simulink model "OLD_slave"  (R2023b)
settings: Solver=VariableStepAuto  StartTime=0.0  StopTime=inf  RelTol=1e-3
settings Model: Creator=sabat  LastModifiedBy=sabat
settings SolverCC: AlgebraicLoopSolver=TrustRegion
settings OptimizationCC: DefaultParameterBehavior=Inlined  EnhancedBackFolding=on  PassReuseOutputArgsAs=Individual arguments  ZeroExternalMemoryAtStartup=off  ZeroInternalMemoryAtStartup=off  OptimizeBlockOrder=speed  DifferentSizesBufferReuse=on  OptimizationCustomize=off  EfficientTunableParamExpr=on
settings DebuggingCC: ParameterTunabilityLossMsg=error
settings SFSimCC: MATLABDynamicMemAlloc=off
settings RTWCC: Description=Embedded Coder  SystemTargetFile=ert.tlc  TemplateMakefile=ert_default_tmf
settings CodeAppCC: ForceParamTrailComments=on  IgnoreCustomStorageClasses=off  OperatorAnnotations=on  SimulinkDataObjDesc=on  SFDataObjDesc=on  InsertBlockDesc=on
settings ERTTargetCC: TargetLangStandard=C99 (ISO)  GenerateSampleERTMain=on  InlinedParameterPlacement=NonHierarchical  ERTCustomFileTemplate=example_file_process.tlc

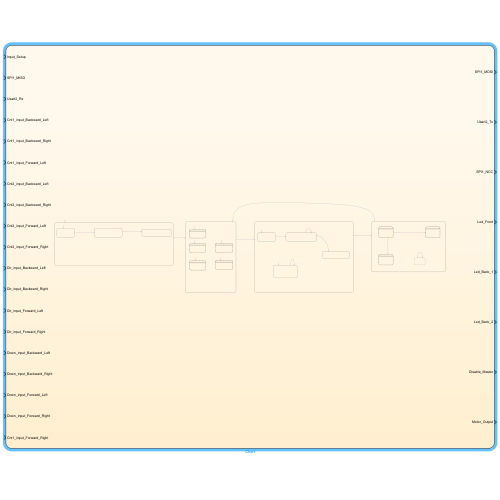
[thumbnail: Simulink's stored preview of the top-level diagram]
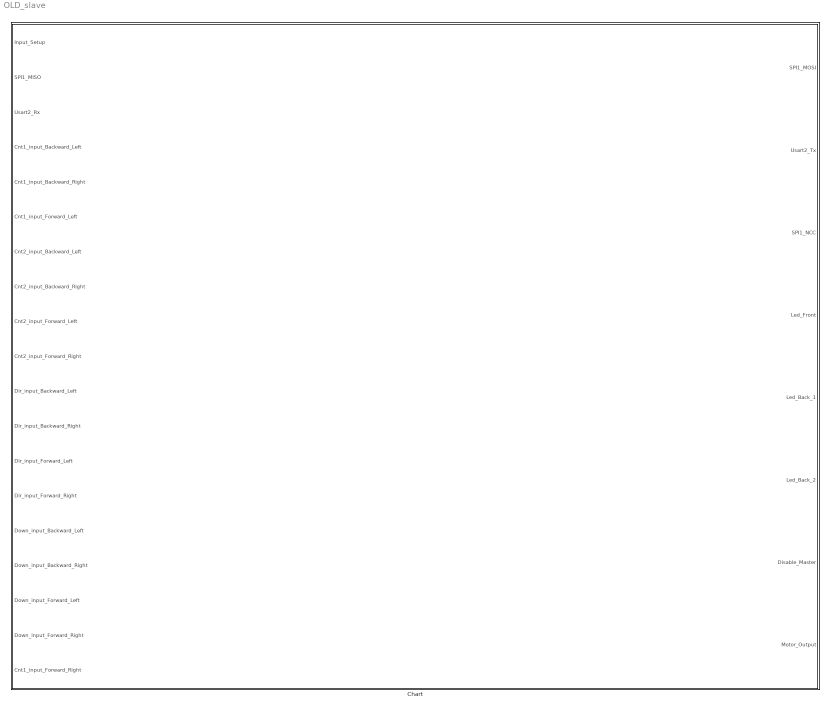
== system OLD_slave ==
  Chart : Stateflow chart  TreatAsAtomicUnit=on

== stateflow chart OLD_slave/Chart ==
  state Read_Inputs_State
    state Logic [parallel]
      settings: executionOrder=1
      state Sensor_Not_Read
      state Sensor_Read
      (default) -> Sensor_Not_Read
      Sensor_Not_Read -> Sensor_Read : [ after(1,Encoder_Backward_Left)   && after(1,Encoder_Backward_Right)  && after(1,Encoder_Forward_Right)  && after(1,Encoder_Forward_Left)  && after(Read_Deadline, msec)]{send(Processing,Read_Inputs_State)}
    state Encoder_Forward_Left [parallel]
      settings: executionOrder=2
      state Read
        cnt2_Forward_Left = Cnt2_input_Forward_Left;
        Dir_Forward_Left = Dir_input_Forward_Left;
        Down_Forward_Left =Down_input_Forward_Left;
        if  Down_Forward_Left
        if (cnt2_Forward_Left < cnt1_Forward_Left)
        diff_Forward_Left = cnt1_Forward_Left - cnt2_Forward_Left;
        else
        diff_Forward_Left = (65535 - cnt2_Forward_Left) + cnt1_Forward_Left;
        end
        else
        if (cnt2_Forward_Left > cnt1_Forward_Left)
        diff _Forward_Left= cnt2_Forward_Left - cnt1_Forward_Left;
        else
        diff _Forward_Left= (65535 - cnt1_Forward_Left) + cnt2_Forward_Left;
        end
        end
        Speed_Forward_Left= diff_Forward_Left / PPR / 60;
      state Start
        cnt1_Forward_Left = Cnt1_input_Forward_Left
      state End
      (default) -> Read_Inputs_State.Encoder_Forward_Left.Start
      Read_Inputs_State.Encoder_Forward_Left.Start -> Read_Inputs_State.Encoder_Forward_Left.Read : [after(300, msec)]
      Read_Inputs_State.Encoder_Forward_Left.Read -> Read_Inputs_State.Encoder_Forward_Left.End : {send(Encoder_Forward_Left,Read_Inputs_State.Logic)}
    state Encoder_Forward_Right [parallel]
      settings: executionOrder=5
      state Read
        cnt2_Forward_Right = Cnt2_input_Forward_Right;
        Dir_Forward_Right = Dir_input_Forward_Right;
        Down_Forward_Right =Down_input_Forward_Right;
        if  Down_Forward_Right
        if (cnt2_Forward_Right < cnt1_Forward_Right)
        diff_Forward_Right = cnt1_Forward_Right - cnt2_Forward_Right;
        else
        diff_Forward_Right = (65535 - cnt2_Forward_Right) + cnt1_Forward_Right;
        end
        else
        if (cnt2_Forward_Right > cnt1_Forward_Right)
        diff _Forward_Right= cnt2_Forward_Right - cnt1_Forward_Right;
        else
        diff _Forward_Right= (65535 - cnt1_Forward_Right) + cnt2_Forward_Right;
        end
        end
        Speed_Forward_Right= diff_Forward_Right / PPR / 60
      state Start
        cnt1_Forward_Right= Cnt1_input_Forward_Right
      state End
      (default) -> Read_Inputs_State.Encoder_Forward_Right.Start
      Read_Inputs_State.Encoder_Forward_Right.Start -> Read_Inputs_State.Encoder_Forward_Right.Read : [after(300, msec)]
      Read_Inputs_State.Encoder_Forward_Right.Read -> Read_Inputs_State.Encoder_Forward_Right.End : {send(Encoder_Forward_Right,Read_Inputs_State.Logic)}
    state Encoder_Backward_Right [parallel]
      settings: executionOrder=4
      state Read
        cnt2_Backward_Right = Cnt2_input_Backward_Right;
        Dir_Backward_Right = Dir_input_Backward_Right;
        Down_Backward_Right =Down_input_Backward_Right;
        if  Down_Backward_Right
        if (cnt2_Backward_Right < cnt1_Backward_Right)
        diff_Backward_Right = cnt1_Backward_Right - cnt2_Backward_Right;
        else
        diff_Backward_Right = (65535 - cnt2_Backward_Right) + cnt1_Backward_Right;
        end
        else
        if (cnt2_Backward_Right > cnt1_Backward_Right)
        diff _Backward_Right= cnt2_Backward_Right - cnt1_Backward_Right;
        else
        diff _Backward_Right= (65535 - cnt1_Backward_Right) + cnt2_Backward_Right;
        end
        end
        Speed_Backward_Right= diff_Backward_Right / PPR / 60
      state Start
        cnt1_Backward_Right= Cnt1_input_Backward_Right
      state End
      (default) -> Read_Inputs_State.Encoder_Backward_Right.Start
      Read_Inputs_State.Encoder_Backward_Right.Start -> Read_Inputs_State.Encoder_Backward_Right.Read : [after(300, msec)]
      Read_Inputs_State.Encoder_Backward_Right.Read -> Read_Inputs_State.Encoder_Backward_Right.End : {send(Encoder_Backward_Right,Read_Inputs_State.Logic)}
    state Encoder_Backward_Left [parallel]
      settings: executionOrder=3
      state Read
        cnt2_Backward_Left = Cnt2_input_Backward_Left;
        Dir_Backward_Left = Dir_input_Backward_Left;
        Down_Backward_Left =Down_input_Backward_Left;
        if  Down_Backward_Left
        if (cnt2_Backward_Left < cnt1_Backward_Left)
        diff_Backward_Left = cnt1_Backward_Left - cnt2_Backward_Left;
        else
        diff_Backward_Left = (65535 - cnt2_Backward_Left) + cnt1_Backward_Left;
        end
        else
        if (cnt2_Backward_Left > cnt1_Backward_Left)
        diff _Backward_Left= cnt2_Backward_Left - cnt1_Backward_Left;
        else
        diff _Backward_Left= (65535 - cnt1_Backward_Left) + cnt2_Backward_Left;
        end
        end
        Speed_Backward_Left= diff_Backward_Left / PPR / 60
      state Start
        cnt1_Backward_Left = Cnt1_input_Backward_Left
      state End
      (default) -> Read_Inputs_State.Encoder_Backward_Left.Start
      Read_Inputs_State.Encoder_Backward_Left.Start -> Read_Inputs_State.Encoder_Backward_Left.Read : [after(300, msec)]
      Read_Inputs_State.Encoder_Backward_Left.Read -> Read_Inputs_State.Encoder_Backward_Left.End : {send(Encoder_Backward_Left,Read_Inputs_State.Logic)}
    (default) -> Logic [order 1]
    (default) -> Encoder_Forward_Left [order 2]
    (default) -> Encoder_Forward_Right [order 4]
    (default) -> Encoder_Backward_Right [order 5]
    (default) -> Encoder_Backward_Left [order 3]
  state Processing_State
    state Read_Master
      Master_Communication = 0;
    state Send_Slave
      en: Global_Struct.Communication="1/2";
      en: Usart2_Tx.Communication=Global_Struct;
    state Go_Other_State
    state Timer_Timer
    Send_Slave -> Send_Slave [order 2] : [after(TIMEOUT,msec)]
    (default) -> Read_Master [order 1]
    Send_Slave -> Go_Other_State [order 1] : [Usart2_Rx.Communication == "Yes"]{
        | Usart2_Tx.Communication ="ACK";
        |  Master_Communication = 1;}
    Read_Master -> Send_Slave : [Usart2_Rx.Communication == "1/2"]
    Timer_Timer -> Timer_Timer : [after(Communication_Deadline, msec)]{send(Outputs,Processing_State)}
    (default) -> Timer_Timer [order 2]
  state Outputs_State
    state Check_Input
      state Check_Board
        if Master_Communication ==1
        ALL_OK = 2;
        else
        ALL_OK=0;
        end
      (default) -> Check_Board
    state Emergency_Stop
      Disable_Master = 1;
      Motor_Output = 0;
    state Attuazione
      state Led
        state LED_Front_OFF
          if Global_Struct.Led_Front == 1
          Led_Front = ~Led_Front;
          end
          if Global_Struct.Led_Back_1 == 1
          Led_Back_1 = ~Led_Back_1;
          end
          if Global_Struct.Led_Back_2 == 1
          Led_Back_2 = ~Led_Back_2;
          end
        (default) -> LED_Front_OFF
      (default) -> Led
    state Timer
    (default) -> Check_Input [order 2]
    Check_Input -> Emergency_Stop [order 2] : [ALL_OK == 2]
    Check_Input -> Attuazione [order 1] : [ALL_OK== 0]
    Timer -> Timer : [after(Outputs_Deadline, msec)]{send(Read_Inputs, Outputs_State)}
    (default) -> Timer [order 1]
  state Setup_State
    state Receive_Master
    state Send_Part
      Usart2_Tx.Communication="Alive";
    state On
      en: send(Read_Inputs,Setup_State);
    (default) -> Receive_Master
    Send_Part -> On : [Input_Setup == 1]
    Receive_Master -> Send_Part : [Usart2_Rx.Communication=="Alive"]
  Outputs_State -> Read_Inputs_State : [Read_Inputs]
  (default) -> Setup_State
  Processing_State -> Outputs_State : [Outputs]
  Setup_State -> Read_Inputs_State : [Read_Inputs]
  Read_Inputs_State -> Processing_State : [Processing]
  data: Input_Setup input double size=1; SPI1_MISO input double size=9; TIMEOUT local double size=1 =15; SPI1_MOSI output double size=[1 2]; Usart2_Tx output Bus: global_var size=1; Usart2_Rx input Bus: global_var size=1; SPI1_NCC output size=1; Global_Struct local Bus: global_var size=1; Led_Front output =0; Led_Back_1 output; Led_Back_2 output; Cnt1_input_Backward_Left input; diff_Backward_Left local; diff_Forward_Left local; diff_Backward_Right local; diff_Forward_Right local; Cnt1_input_Backward_Right input; Cnt1_input_Forward_Left input; Cnt2_input_Backward_Left input; Cnt2_input_Backward_Right input; Cnt2_input_Forward_Left input; Cnt2_input_Forward_Right input; Dir_input_Backward_Left input; Dir_input_Backward_Right input; Dir_input_Forward_Left input; Dir_input_Forward_Right input; Down_input_Backward_Left input; Down_input_Backward_Right input; Down_input_Forward_Left input; Down_input_Forward_Right input; Cnt1_input_Forward_Right input; Dir_Backward_Left local; Dir_Backward_Right local; Dir_Forward_Left local; Dir_Forward_Right local; Down_Forward_Left local; Down_Forward_Right local; cnt1_Backward_Right local; cnt1_Forward_Right local; cnt1_Backward_Left local; cnt2_Backward_Left local; cnt2_Forward_Left local; cnt2_Forward_Right local; Down_Backward_Left local; cnt1_Forward_Left local; cnt2_Backward_Right local; ALL_OK local; Down_Backward_Right local; Master_Communication local; Communication_Deadline local =50; Read_Deadline local =50; Outputs_Deadline local =50; Disable_Master output; Speed_Backward_Left local; Speed_Backward_Right local; Speed_Forward_Left local; Speed_Forward_Right local; PPR local =12; Motor_Output output
  events: Processing local FUNCTION_CALL_EVENT; Read_Inputs local FUNCTION_CALL_EVENT; Outputs local FUNCTION_CALL_EVENT; Encoder_Backward_Left local FUNCTION_CALL_EVENT; Encoder_Forward_Left local FUNCTION_CALL_EVENT; Encoder_Backward_Right local FUNCTION_CALL_EVENT; Encoder_Forward_Right local FUNCTION_CALL_EVENT
